simulink model "pendulum_rwp_v2"  (R2022a)
settings: Solver=VariableStepAuto  StartTime=0.0  StopTime=10  MaxStep=0.01  RelTol=1e-3  EnableMultiTasking=on
values from neighbouring files (symbols this model uses):
  A = [0 1 0 0; (b*g)/(a-J2) -c1/(a-J2) 0 c2/(a-J2); 0 0 0 1; -(b*g)/(a-J2) c1/(a-J2) 0 (a*c2)/(J2*(a-J2))]    [simulate_the_effect_of_inertia_moment_j2.m]
  a = m1*l1^2 + m1*l2^2 + J1 + J2    (= 0.07321486234)    [simulate_the_effect_of_inertia_moment_j2.m]
  B = [0; 1/(a-J2); 0; a/(J2*(a-J2))]    [simulate_the_effect_of_inertia_moment_j2.m]
  b = m1*l1 + m2*l2    (= 0.2327278)    [simulate_the_effect_of_inertia_moment_j2.m]
  c1 = 0.04    [simulate_the_effect_of_inertia_moment_j2.m]
  c2 = 0.0001    [simulate_the_effect_of_inertia_moment_j2.m]
  g = 9.82    [simulate_the_effect_of_inertia_moment_j2.m]
  J2 = 0.005    [simulate_the_effect_of_inertia_moment_j2.m]
  K = acker(A, B, p)    [simulate_the_effect_of_inertia_moment_j2.m]
  Kb = 0.0987    [simulate_the_effect_of_inertia_moment_j2.m]
  Kt = 0.0987    [simulate_the_effect_of_inertia_moment_j2.m]
  Ra = 1.556    [simulate_the_effect_of_inertia_moment_j2.m]
  theta_0 = 0.0349    [simulate_the_effect_of_inertia_moment_j2.m]
undefined symbols (not defined in the file or in its folder): C1, C2, D, x0
libraries: simulink_extras x2
Description:
  | modified 22.10.2021
settings Model: Creator=TL RT-Lab  LastModifiedBy=mchae
settings Model: ModifiedHistory=|
  | init: Okt. 2021
  | current version v2
settings SolverCC: AlgebraicLoopSolver=TrustRegion
settings DataIOCC: SaveFormat=Array  SaveOutput=off  SignalLogging=off  DSMLogging=off  SaveTime=off  ReturnWorkspaceOutputs=off
settings OptimizationCC: OptimizeBlockIOStorage=off  BufferReuse=off  GlobalBufferReuse=off  ExpressionFolding=off  LocalBlockOutputs=off  LifeSpan=inf
settings DebuggingCC: SolverPrmCheckMsg=warning  UnconnectedInputMsg=warning  UnconnectedOutputMsg=warning  UnconnectedLineMsg=warning  AllowSymbolicDim=off  SFUnexpectedBacktrackingDiag=warning  SFNoUnconditionalDefaultTransitionDiag=warning  SFExecutionAtInitializationDiag=none  SFMachineParentedDataDiag=warning  ArithmeticOperatorsInVariantConditions=warning
settings HardwareCC: ProdBitPerPointer=32  ProdBitPerSizeT=32  ProdBitPerPtrDiffT=32  ProdLargestAtomicFloat=None  ProdIntDivRoundTo=Undefined  ProdEndianess=Unspecified  ProdWordSize=32  ProdHWDeviceType=32-bit Generic
settings ModelReferenceCC: PropagateSignalLabelsOutOfModel=off
settings SFSimCC: SimUseLocalCustomCode=off  CustomCodeUndefinedFunction=UseInterfaceOnly
settings RTWCC: RTWUseLocalCustomCode=off  DLArmComputeVersion=19.05
settings CodeAppCC: StateflowObjectComments=on
settings GRTTargetCC: TargetLangStandard=C89/C90 (ANSI)
settings ConfigComp: CovMetricSettings=dw  CovSaveCumulativeToWorkspaceVar=on  CovSaveSingleToWorkspaceVar=on  CovExternalEMLEnable=off

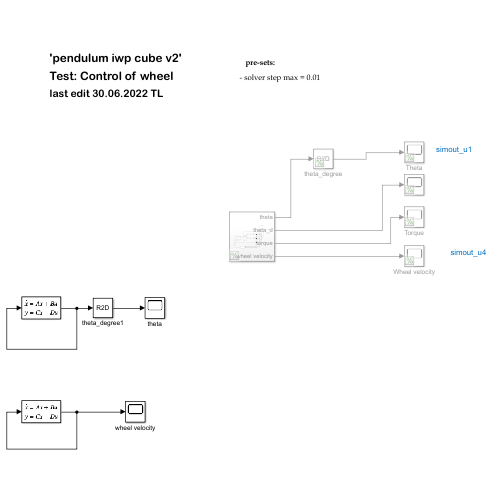
[thumbnail: Simulink's stored preview of the top-level diagram]
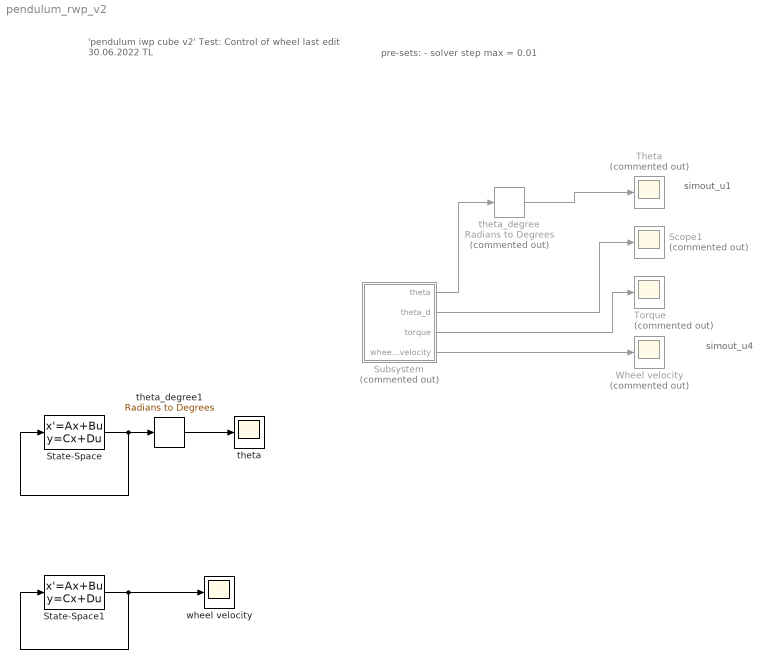
== system pendulum_rwp_v2 ==
  note: 'pendulum iwp cube v2'
      |
      | Test: Control of wheel
      |
      | last edit 30.06.2022 TL
  note: pre-sets:
      |
      | - solver step max = 0.01
  note: simout_u1
  note: simout_u4
  Scope1 : Scope  Commented=on
  State-Space : StateSpace  A=A-B*K  B=B  C=C1  D=D  InitialCondition=x0
  State-Space1 : StateSpace  A=A-B*K  B=B  C=C2  D=D  InitialCondition=x0
  Subsystem : Subsystem  Commented=on
  Theta : Scope  Commented=on
  Torque : Scope  Commented=on
  Wheel velocity : Scope  Commented=on
  theta : Scope
  theta_degree : simulink_extras/Transformations/Radians to Degrees  Commented=on
  theta_degree1 : simulink_extras/Transformations/Radians to Degrees
  wheel velocity : Scope
  wires:
  theta_degree/1 -> Theta/1
  Subsystem/1(theta) -> theta_degree/1
  Subsystem/2(theta_d) -> Scope1/1
  Subsystem/3(torque) -> Torque/1
  Subsystem/4(wheel velocity) -> Wheel velocity/1
  State-Space/1 -> theta_degree1/1, State-Space/1
  State-Space1/1 -> wheel velocity/1, State-Space1/1
  theta_degree1/1 -> theta/1

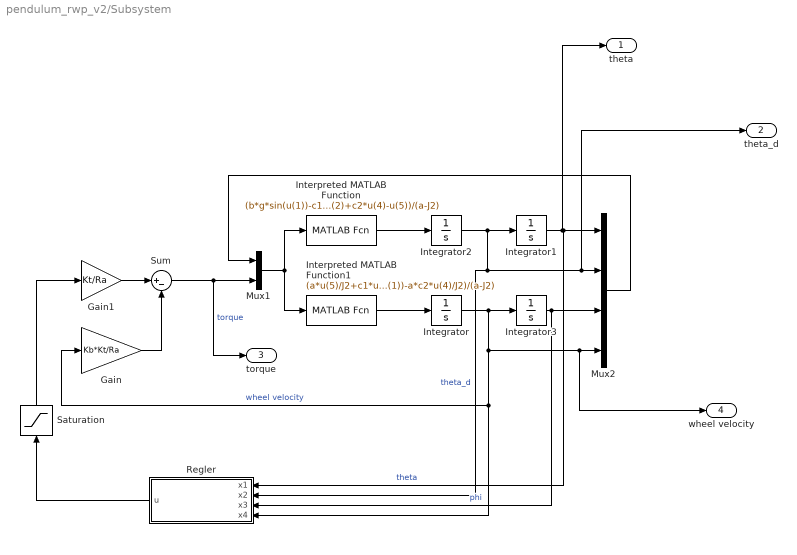
== system pendulum_rwp_v2/Subsystem ==
  Gain : Gain  Gain=Kb*Kt/Ra
  Gain1 : Gain  Gain=Kt/Ra
  Integrator : Integrator
  Integrator1 : Integrator  InitialCondition=theta_0
  Integrator2 : Integrator
  Integrator3 : Integrator
  Interpreted MATLAB Function : MATLABFcn  MATLABFcn=(b*g*sin(u(1))-c1*u(2)+c2*u(4)-u(5))/(a-J2)  Output1D=off
  Interpreted MATLAB Function1 : MATLABFcn  MATLABFcn=(a*u(5)/J2+c1*u(2)-b*g*sin(u(1))-a*c2*u(4)/J2)/(a-J2)  Output1D=off
  Mux1 : Mux  Inputs=2
  Mux2 : Mux
  Regler : Subsystem
  Saturation : Saturate  UpperLimit=30  LowerLimit=-30
  Sum : Sum  Inputs=|+-
  theta : Outport
  theta_d : Outport  Port=2
  torque : Outport  Port=3
  wheel velocity : Outport  Port=4
  wires:
  Integrator1/1 -> theta/1, Mux2/1, Regler/1(x1)  "theta"
  Integrator2/1 -> Integrator1/1, Regler/2(x2), theta_d/1, Mux2/2  "theta_d"
  Integrator3/1 -> Regler/3(x3), Mux2/3  "phi"
  Gain/1 -> Sum/2
  Mux2/1 -> Mux1/1
  Sum/1 -> torque/1, Mux1/2  "torque"
  Integrator/1 -> Regler/4(x4), Gain/1, wheel velocity/1, Mux2/4, Integrator3/1  "wheel velocity"
  Interpreted MATLAB Function/1 -> Integrator2/1
  Interpreted MATLAB Function1/1 -> Integrator/1
  Regler/1(u) -> Saturation/1
  Gain1/1 -> Sum/1
  Mux1/1 -> Interpreted MATLAB Function1/1, Interpreted MATLAB Function/1
  Saturation/1 -> Gain1/1

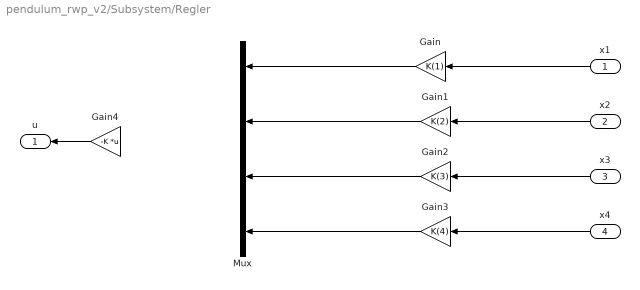
== system pendulum_rwp_v2/Subsystem/Regler ==
  x1 : Inport
  x2 : Inport  Port=2
  x3 : Inport  Port=3
  x4 : Inport  Port=4
  Gain : Gain  Gain=K(1)
  Gain1 : Gain  Gain=K(2)
  Gain2 : Gain  Gain=K(3)
  Gain3 : Gain  Gain=K(4)
  Gain4 : Gain  Gain=-K  Multiplication=Matrix(K*u)
  Mux : Mux
  u : Outport
  wires:
  x1/1 -> Gain/1
  x2/1 -> Gain1/1
  x3/1 -> Gain2/1
  x4/1 -> Gain3/1
  ? -> Gain4/1
  Gain4/1 -> u/1
  Gain/1 -> Mux/1
  Gain3/1 -> Mux/4
  Gain2/1 -> Mux/3
  Gain1/1 -> Mux/2
